simulink model "unitTestSLoWC"  (R2018b)
settings: Solver=VariableStepAuto  StartTime=0.0  StopTime=10.0  RelTol=1e-3
libraries: SLoWCBlock x1
settings Model: Creator=PE29732  LastModifiedBy=BI28030

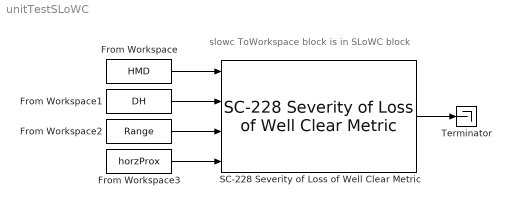
== system unitTestSLoWC ==
  note: slowc ToWorkspace block is in SLoWC block
  From Workspace : FromWorkspace  VariableName=HMD  SampleTime=0
  From Workspace1 : FromWorkspace  VariableName=DH  SampleTime=0
  From Workspace2 : FromWorkspace  VariableName=Range  SampleTime=0
  From Workspace3 : FromWorkspace  VariableName=horzProx  SampleTime=0
  SC-228 Severity of Loss of Well Clear Metric : SLoWCBlock/SC-228 Severity of Loss of Well Clear Metric  DMOD=4000  altDiffThreshold=450
  Terminator : Terminator
  wires:
  SC-228 Severity of Loss of Well Clear Metric/1 -> Terminator/1
  From Workspace/1 -> SC-228 Severity of Loss of Well Clear Metric/1
  From Workspace1/1 -> SC-228 Severity of Loss of Well Clear Metric/2
  From Workspace2/1 -> SC-228 Severity of Loss of Well Clear Metric/3
  From Workspace3/1 -> SC-228 Severity of Loss of Well Clear Metric/4
